simulink model "demostration3"  (R2014b)
settings: Solver=ode45  StartTime=0.0  StopTime=60  RelTol=1e-3
settings Model: Creator=wangze  LastModifiedBy=wangze
settings DataIOCC: LimitDataPoints=off
settings OptimizationCC: UseDivisionForNetSlopeComputation=off  SimCompilerOptimization=off
settings DebuggingCC: FrameProcessingCompatibilityMsg=error  AllowSymbolicDim=off
settings RTWCC: RTWCompilerOptimization=off
settings ConfigComp: CovMetricSettings=dw  CovHtmlReporting=on  CovSaveCumulativeToWorkspaceVar=on  CovSaveSingleToWorkspaceVar=on  CovModelRefEnable=Off  CovExternalEMLEnable=off  CovSFcnEnable=off

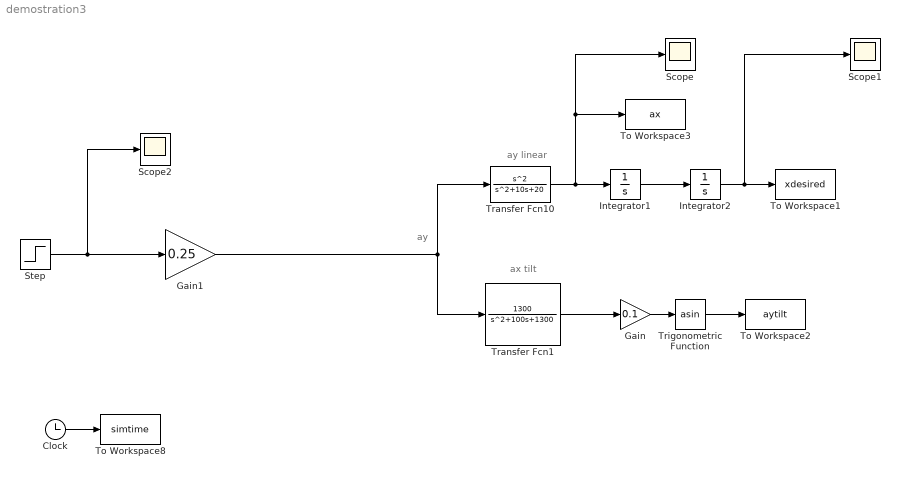
== system demostration3 ==
  note: ax tilt
  note: ay linear
  note: ay
  Clock : Clock
  Gain : Gain  Gain=0.1
  Gain1 : Gain  Gain=0.25
  Integrator1 : Integrator
  Integrator2 : Integrator
  Scope : Scope
  Scope1 : Scope
  Scope2 : Scope
      settings: SaveName=ScopeData2
  Step : Step  Time=0  After=9.8  SampleTime=0.05
  To Workspace1 : ToWorkspace  VariableName=xdesired  SampleTime=-1
  To Workspace2 : ToWorkspace  VariableName=aytilt  SampleTime=-1
  To Workspace3 : ToWorkspace  VariableName=ax  SampleTime=-1
  To Workspace8 : ToWorkspace  VariableName=simtime  SampleTime=-1
      settings: Decimation=2  Save2DSignal=2-D array (concatenate along first dimension)
  Transfer Fcn1 : TransferFcn  Numerator=[1300]  Denominator=[1 100 1300]
  Transfer Fcn10 : TransferFcn  Numerator=[1 0 0]  Denominator=[1 10 20]
  Trigonometric Function : Trigonometry  Operator=asin
  wires:
  Gain1/1 -> Transfer Fcn1/1, Transfer Fcn10/1
  Transfer Fcn10/1 -> Scope/1, To Workspace3/1, Integrator1/1
  Integrator1/1 -> Integrator2/1
  Integrator2/1 -> Scope1/1, To Workspace1/1
  Transfer Fcn1/1 -> Gain/1
  Gain/1 -> Trigonometric Function/1
  Trigonometric Function/1 -> To Workspace2/1
  Clock/1 -> To Workspace8/1
  Step/1 -> Scope2/1, Gain1/1
